simulink model "simulinkProject"  (R2023a)
settings: Solver=ode4  StartTime=0.0  StopTime=20  FixedStep=System.Ts  RelTol=1e-3
values from neighbouring files (symbols this model uses):
  b_end = 0.5*(K_end * (Lift.m + Tilt.m + Cylinder_3.m + Extension_2.m + Extension_1.m + Cylinder_4.m))^0.5    [project.m]
  b_end_1 = 0.5*(K_end_1 * (Lift.m + Pillar.m + Cylinder.m + Tilt.m + Cylinder_4.m + Cylinder_3.m + Extension_1.m + Extension_2.m))^0.5    [project.m]
  b_end_3 = 0.5*(K_end_3 * (Tilt.m + Extension_2.m + Extension_1.m + Cylinder_4.m))^0.5    [project.m]
  b_end_4 = 0.5*(K_end_4 * (Extension_2.m + Extension_1.m))^0.5    [project.m]
  K_end = p_max / delta_x    [project.m]
  K_end_1 = p_max_1 / delta_x_1    [project.m]
  K_end_3 = p_max_3 / delta_x_3    [project.m]
  K_end_4 = p_max_4 / delta_x_4    [project.m]
  Offset = 0.92    [project.m]
  Offset_1 = 0.72    [project.m]
  Offset_4 = 2.640    (= 2.64)    [project.m]
undefined symbols (not defined in the file or in its folder): Cylinder, Cylinder_1, Cylinder_3, Cylinder_4, Extension_1, fabs, Fourbar_1, Fourbar_2, Lift, Pillar, Pinion, Piston, Piston_3, Piston_4, sgn, System, System_1, System_3, System_4, Tilt, Valve, Valve_1, Valve_3, Valve_4, X, Y, Z
libraries: sm_lib x71, nesl_utility x27, TcTargetLib x1
(part 2 of 4)

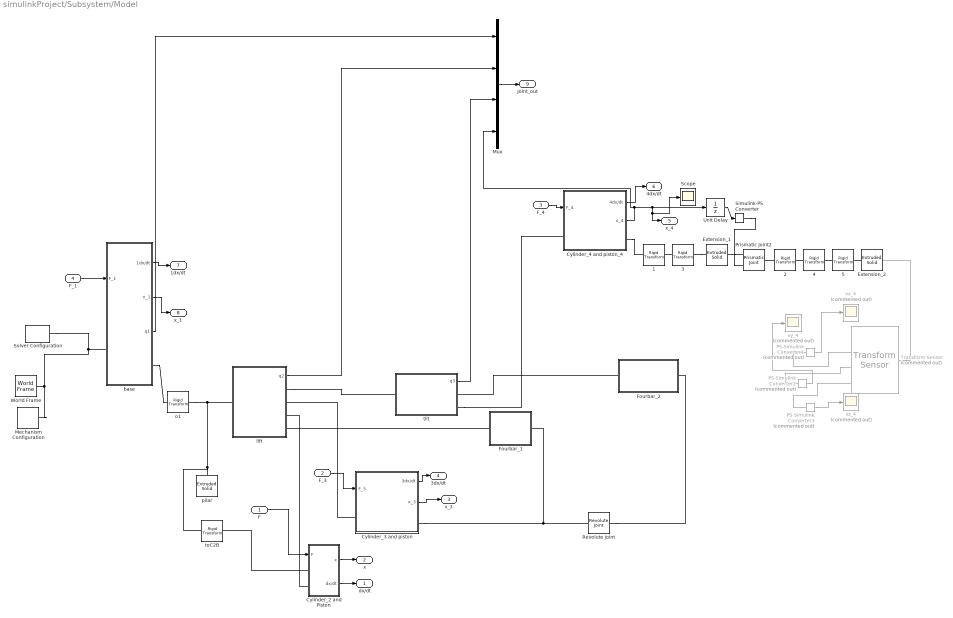
== system simulinkProject/Subsystem/Model ==
  F : Inport
  F_3 : Inport  Port=2
  F_4 : Inport  Port=3
  F_1 : Inport  Port=4
  1 : sm_lib/Frames and Transforms/Rigid Transform  TranslationMethod=None  TranslationStandardOffset=-0.2  TranslationStandardOffsetUnits=m  TranslationStandardAxis=+X  TranslationCartesianOffset=[0 0 -0.177]  TranslationCartesianOffsetUnits=m  TranslationROffset=0  TranslationROffsetUnits=m  TranslationZOffset=0  TranslationZOffsetUnits=m  TranslationThetaOffset=0  TranslationThetaOffsetUnits=deg  RotationMethod=StandardAxis  RotationAngleUnits=deg  RotationStandardAxis=-Y  RotationAngle=90.0  RotationArbitraryAxis=[0 0 1]  FollAlignAxisA=+X  BaseAlignAxisA=+Y  FollAlignAxisB=+Y  BaseAlignAxisB=+Z  RotationSequenceAxes=FollowerAxes  RotationSequence=XYX  RotationSequenceAngles=[0 0 0]  RotationSequenceAnglesUnits=deg  RotationMatrix=[1 0 0; 0 1 0; 0 0 1]  Quaternion=[1 0 0 0]
  2 : sm_lib/Frames and Transforms/Rigid Transform  TranslationMethod=None  TranslationStandardOffset=-0.5  TranslationStandardOffsetUnits=m  TranslationStandardAxis=-Z  TranslationCartesianOffset=[0 0 -0.177]  TranslationCartesianOffsetUnits=m  TranslationROffset=0  TranslationROffsetUnits=m  TranslationZOffset=0  TranslationZOffsetUnits=m  TranslationThetaOffset=0  TranslationThetaOffsetUnits=deg  RotationMethod=None  RotationAngleUnits=deg  RotationStandardAxis=+Y  RotationAngle=90.0  RotationArbitraryAxis=[0 0 1]  FollAlignAxisA=+X  BaseAlignAxisA=+Y  FollAlignAxisB=+Y  BaseAlignAxisB=+Z  RotationSequenceAxes=FollowerAxes  RotationSequence=XYX  RotationSequenceAngles=[0 0 0]  RotationSequenceAnglesUnits=deg  RotationMatrix=[1 0 0; 0 1 0; 0 0 1]  Quaternion=[1 0 0 0]
  3 : sm_lib/Frames and Transforms/Rigid Transform  TranslationMethod=None  TranslationStandardOffset=-0.2  TranslationStandardOffsetUnits=m  TranslationStandardAxis=+X  TranslationCartesianOffset=[0 0 -0.177]  TranslationCartesianOffsetUnits=m  TranslationROffset=0  TranslationROffsetUnits=m  TranslationZOffset=0  TranslationZOffsetUnits=m  TranslationThetaOffset=0  TranslationThetaOffsetUnits=deg  RotationMethod=StandardAxis  RotationAngleUnits=deg  RotationStandardAxis=-X  RotationAngle=90.0  RotationArbitraryAxis=[0 0 1]  FollAlignAxisA=+X  BaseAlignAxisA=+Y  FollAlignAxisB=+Y  BaseAlignAxisB=+Z  RotationSequenceAxes=FollowerAxes  RotationSequence=XYX  RotationSequenceAngles=[0 0 0]  RotationSequenceAnglesUnits=deg  RotationMatrix=[1 0 0; 0 1 0; 0 0 1]  Quaternion=[1 0 0 0]
  4 : sm_lib/Frames and Transforms/Rigid Transform  TranslationMethod=None  TranslationStandardOffset=-0.2  TranslationStandardOffsetUnits=m  TranslationStandardAxis=+X  TranslationCartesianOffset=[0 0 -0.177]  TranslationCartesianOffsetUnits=m  TranslationROffset=0  TranslationROffsetUnits=m  TranslationZOffset=0  TranslationZOffsetUnits=m  TranslationThetaOffset=0  TranslationThetaOffsetUnits=deg  RotationMethod=StandardAxis  RotationAngleUnits=deg  RotationStandardAxis=+X  RotationAngle=90.0  RotationArbitraryAxis=[0 0 1]  FollAlignAxisA=+X  BaseAlignAxisA=+Y  FollAlignAxisB=+Y  BaseAlignAxisB=+Z  RotationSequenceAxes=FollowerAxes  RotationSequence=XYX  RotationSequenceAngles=[0 0 0]  RotationSequenceAnglesUnits=deg  RotationMatrix=[1 0 0; 0 1 0; 0 0 1]  Quaternion=[1 0 0 0]
  5 : sm_lib/Frames and Transforms/Rigid Transform  TranslationMethod=None  TranslationStandardOffset=-0.2  TranslationStandardOffsetUnits=m  TranslationStandardAxis=+X  TranslationCartesianOffset=[0 0 -0.177]  TranslationCartesianOffsetUnits=m  TranslationROffset=0  TranslationROffsetUnits=m  TranslationZOffset=0  TranslationZOffsetUnits=m  TranslationThetaOffset=0  TranslationThetaOffsetUnits=deg  RotationMethod=StandardAxis  RotationAngleUnits=deg  RotationStandardAxis=-X  RotationAngle=90.0  RotationArbitraryAxis=[0 0 1]  FollAlignAxisA=+X  BaseAlignAxisA=+Y  FollAlignAxisB=+Y  BaseAlignAxisB=+Z  RotationSequenceAxes=FollowerAxes  RotationSequence=XYX  RotationSequenceAngles=[0 0 0]  RotationSequenceAnglesUnits=deg  RotationMatrix=[1 0 0; 0 1 0; 0 0 1]  Quaternion=[1 0 0 0]
  Cylinder_2 and Piston : Subsystem
  Cylinder_3 and piston : Subsystem
  Cylinder_4 and piston_4 : Subsystem
  Extension_1 : sm_lib/Body Elements/Extruded Solid  GraphicAmbientColor=[0.15 0.15 0.15 1.0]  BasedOnType=Mass  CenterOfMass=Extension_1.cm  CenterOfMassUnits=m  GraphicDiffuseColor=[0.0 0.6 0.6]  ExportConvexHullGeometry=off  ExtrusionCrossSection=Extension_1.cs  ExtrusionCrossSectionUnits=m  Density=1000  DensityUnits=kg/m^3  DoExposeReferenceFrame=off  GraphicEmissiveColor=[0.0 0.0 0.0 1.0]  ExportEntireGeometry=off  ExtrusionLength=0.2  ExtrusionLengthUnits=m  ExtrusionType=General  SerializedFrames=<Frames><Frame><Id>Frame1</Id><Value><Name>F1</Name><Origin><Source>GeometricFeature</Source><FeatureName>side surface 6</FeatureName></Origin><PrimaryAxis><DefinedDirection>+Z</DefinedDirection><Source>ReferenceFrame</Source><SourceDirection>+X</SourceDirection><FeatureName></FeatureName></PrimaryAxis><SecondaryAxis><DefinedDirection>+X</DefinedDirection><Source>ReferenceFrame</Source><SourceDirection>+Y</SourceDirection><FeatureName></FeatureName></SecondaryAxis></Value></Frame><Frame><Id>Frame2</Id><Value><Name>F2</Name><Origin><Source>GeometricFeature</Source><FeatureName>side curve 3</FeatureName></Origin><PrimaryAxis><DefinedDirection>+Z</DefinedDirection><Source>ReferenceFrame</Source><SourceDirection>+Z</SourceDirection><FeatureName></FeatureName></PrimaryAxis><SecondaryAxis><DefinedDirection>+X</DefinedDirection><Source>ReferenceFrame</Source><SourceDirection>+X</SourceDirection><FeatureName></FeatureName></SecondaryAxis></Value></Frame></Frames>  MarkerShape=Sphere  MarkerSize=10  GraphicType=FromGeometry  InertiaType=CalculateFromGeometry  Mass=Extension_1.m  MassUnits=kg  MomentsOfInertia=[1 1 1]  MomentsOfInertiaUnits=kg*m^2  PolygonNumSides=3  GraphicOpacity=1.0  PolygonOuterRadius=1  PolygonOuterRadiusUnits=m  ProductsOfInertia=[0 0 0]  ProductsOfInertiaUnits=kg*m^2  GraphicShininess=75  GraphicSpecularColor=[0.5 0.5 0.5 1.0]  GraphicVisPropType=SimpleVisualProperties
  Extension_2 : sm_lib/Body Elements/Extruded Solid  GraphicAmbientColor=[0.15 0.15 0.15 1.0]  BasedOnType=Mass  CenterOfMass=Extension_1.cm  CenterOfMassUnits=m  GraphicDiffuseColor=[0.2 0.0 0.4]  ExportConvexHullGeometry=off  ExtrusionCrossSection=Extension_1.cs  ExtrusionCrossSectionUnits=m  Density=1000  DensityUnits=kg/m^3  DoExposeReferenceFrame=off  GraphicEmissiveColor=[0.0 0.0 0.0 1.0]  ExportEntireGeometry=off  ExtrusionLength=0.2  ExtrusionLengthUnits=m  ExtrusionType=General  SerializedFrames=<Frames><Frame><Id>Frame1</Id><Value><Name>F1</Name><Origin><Source>GeometricFeature</Source><FeatureName>side surface 6</FeatureName></Origin><PrimaryAxis><DefinedDirection>+Z</DefinedDirection><Source>ReferenceFrame</Source><SourceDirection>+X</SourceDirection><FeatureName></FeatureName></PrimaryAxis><SecondaryAxis><DefinedDirection>+X</DefinedDirection><Source>ReferenceFrame</Source><SourceDirection>+Y</SourceDirection><FeatureName></FeatureName></SecondaryAxis></Value></Frame><Frame><Id>Frame2</Id><Value><Name>F2</Name><Origin><Source>GeometricFeature</Source><FeatureName>side curve 3</FeatureName></Origin><PrimaryAxis><DefinedDirection>+Z</DefinedDirection><Source>ReferenceFrame</Source><SourceDirection>+Z</SourceDirection><FeatureName></FeatureName></PrimaryAxis><SecondaryAxis><DefinedDirection>+X</DefinedDirection><Source>ReferenceFrame</Source><SourceDirection>+X</SourceDirection><FeatureName></FeatureName></SecondaryAxis></Value></Frame></Frames>  MarkerShape=Sphere  MarkerSize=10  GraphicType=FromGeometry  InertiaType=CalculateFromGeometry  Mass=Extension_1.m  MassUnits=kg  MomentsOfInertia=[1 1 1]  MomentsOfInertiaUnits=kg*m^2  PolygonNumSides=3  GraphicOpacity=1.0  PolygonOuterRadius=1  PolygonOuterRadiusUnits=m  ProductsOfInertia=[0 0 0]  ProductsOfInertiaUnits=kg*m^2  GraphicShininess=75  GraphicSpecularColor=[0.5 0.5 0.5 1.0]  GraphicVisPropType=SimpleVisualProperties
  Fourbar_1 : Subsystem
  Fourbar_2 : Subsystem
  Mechanism Configuration : sm_lib/Utilities/Mechanism Configuration  UniformGravity=Constant  GravityVector=[0 0 -9.80665]  GravityVectorUnits=m/s^2  LinearizationDelta=0.001  JointModeTransitionNonlinearIterations=2
  Mux : Mux
  PS-Simulink Converter1 : nesl_utility/PS-Simulink Converter  Commented=on  PhysicalDomain=network_engine_domain  SubClassName=ps_output  LeftPortType=input  RightPortType=output  PseudoPeriodic=off  Frequencies=[]  VectorFormat=inherit  Unit=inherit  AffineConversion=off
  PS-Simulink Converter2 : nesl_utility/PS-Simulink Converter  Commented=on  PhysicalDomain=network_engine_domain  SubClassName=ps_output  LeftPortType=input  RightPortType=output  PseudoPeriodic=off  Frequencies=[]  VectorFormat=inherit  Unit=inherit  AffineConversion=off
  PS-Simulink Converter3 : nesl_utility/PS-Simulink Converter  Commented=on  PhysicalDomain=network_engine_domain  SubClassName=ps_output  LeftPortType=input  RightPortType=output  PseudoPeriodic=off  Frequencies=[]  VectorFormat=inherit  Unit=inherit  AffineConversion=off
  Prismatic Joint2 : sm_lib/Joints/Prismatic Joint  JointMode=Normal  SenseConstraintForce=off  SenseConstraintForceX=off  SenseConstraintForceY=off  SenseConstraintForceZ=off  SenseConstraintTorque=off  SenseConstraintTorqueX=off  SenseConstraintTorqueY=off  SenseConstraintTorqueZ=off  SenseTotalForce=off  SenseTotalForceX=off  SenseTotalForceY=off  SenseTotalForceZ=off  SenseTotalTorque=off  SenseTotalTorqueX=off  SenseTotalTorqueY=off  SenseTotalTorqueZ=off  CompositeWrenchDir=FollowerOnBase  CompositeWrenchFrame=BaseFrame  EquilibriumPosition=0  EquilibriumPositionUnits=m  SpringStiffness=0  SpringStiffnessUnits=N/m  DampingCoefficient=0  DampingCoefficientUnits=N/(m/s)  TorqueActuationMode=ComputedTorque  MotionActuationMode=InputMotion  SensePosition=off  SenseVelocity=off  SenseAcceleration=off  SenseTorqueForce=off  SenseLowerLimitTorqueForce=off  SenseUpperLimitTorqueForce=off  LowerLimitSpecify=off  LowerLimitBound=-1  LowerLimitBoundUnits=m  LowerLimitStiffness=1e6  LowerLimitStiffnessUnits=N/m  LowerLimitDamping=1e3  LowerLimitDampingUnits=N/(m/s)  LowerLimitTransitionRegionWidth=1e-4  LowerLimitTransitionRegionWidthUnits=m  UpperLimitSpecify=off  UpperLimitBound=1  UpperLimitBoundUnits=m  UpperLimitStiffness=1e6  UpperLimitStiffnessUnits=N/m  UpperLimitDamping=1e3  UpperLimitDampingUnits=N/(m/s)  UpperLimitTransitionRegionWidth=1e-4  UpperLimitTransitionRegionWidthUnits=m  PositionTargetSpecify=on  PositionTargetPriority=High  PositionTargetValue=0.2  PositionTargetValueUnits=m  VelocityTargetSpecify=off  VelocityTargetPriority=High  VelocityTargetValue=0  VelocityTargetValueUnits=m/s
  Revolute Joint : sm_lib/Joints/Revolute Joint  JointMode=Normal  SenseConstraintForce=off  SenseConstraintForceX=off  SenseConstraintForceY=off  SenseConstraintForceZ=off  SenseConstraintTorque=off  SenseConstraintTorqueX=off  SenseConstraintTorqueY=off  SenseConstraintTorqueZ=off  SenseTotalForce=off  SenseTotalForceX=off  SenseTotalForceY=off  SenseTotalForceZ=off  SenseTotalTorque=off  SenseTotalTorqueX=off  SenseTotalTorqueY=off  SenseTotalTorqueZ=off  CompositeWrenchDir=FollowerOnBase  CompositeWrenchFrame=BaseFrame  EquilibriumPosition=0  EquilibriumPositionUnits=deg  SpringStiffness=0  SpringStiffnessUnits=N*m/deg  DampingCoefficient=0  DampingCoefficientUnits=N*m/(deg/s)  TorqueActuationMode=NoTorque  MotionActuationMode=ComputedMotion  SensePosition=off  SenseVelocity=off  SenseAcceleration=off  SenseTorqueForce=off  SenseLowerLimitTorqueForce=off  SenseUpperLimitTorqueForce=off  LowerLimitSpecify=off  LowerLimitBound=-90  LowerLimitBoundUnits=deg  LowerLimitStiffness=1e4  LowerLimitStiffnessUnits=N*m/deg  LowerLimitDamping=10  LowerLimitDampingUnits=N*m/(deg/s)  LowerLimitTransitionRegionWidth=0.1  LowerLimitTransitionRegionWidthUnits=deg  UpperLimitSpecify=off  UpperLimitBound=90  UpperLimitBoundUnits=deg  UpperLimitStiffness=1e4  UpperLimitStiffnessUnits=N*m/deg  UpperLimitDamping=10  UpperLimitDampingUnits=N*m/(deg/s)  UpperLimitTransitionRegionWidth=0.1  UpperLimitTransitionRegionWidthUnits=deg  PositionTargetSpecify=off  PositionTargetPriority=Low  PositionTargetValue=-80  PositionTargetValueUnits=deg  VelocityTargetSpecify=off  VelocityTargetPriority=High  VelocityTargetValue=0  VelocityTargetValueUnits=deg/s
  Scope : Scope
  Simulink-PS Converter : nesl_utility/Simulink-PS Converter  PhysicalDomain=network_engine_domain  SubClassName=ps_input  LeftPortType=input  RightPortType=output  PseudoPeriodic=off  Frequencies=[]  NoiseDistribution=none  NoiseParameters=[]  Unit=1  AffineConversion=off  FilteringAndDerivatives=filter  SimscapeFilterOrder=2  InputFilterTimeConstant=0.005  UdotUserProvided=0
  Solver Configuration : nesl_utility/Solver Configuration  PhysicalDomain=network_engine_domain  SubClassName=solver  LeftPortType=input  RightPortType=generic  Tones=[]  Harmonics=[]  SimulateNoise=off  Profile=off  UseLocalSampling=off  EnableSwitchedLinearOptims=on  FrequencyDomain=off  UseCCode=off  RelTol=0.001  AbsTol=0.001  MinStep=1e-09  ToWorkspace=off  RevertToSquareIcSolve=off  NumHomotopyIterations=100  PhasorMode=off  PhasorModeNumHarmonics=1  ConsistencySolver=NEWTON_XTOL_AFTER_FTOL  IndexReductionMethod=DerivativeReplacement  DoDC=off  ResidualTolerance=1e-09  ConsistencyTolSource=GLOBAL  ConsistencyAbsTol=0.001  ConsistencyRelTol=0.001  ConsistencyTolFactor=0.001  UseLocalSolver=off  LocalSolverChoice=NE_BACKWARD_EULER_ADVANCER  ResolveIndetEquations=on  FunctionEvalNumThread=1  LocalSolverSampleTime=0.001  DoFixedCost=off  MaxNonlinIter=3  MaxModeIter=2  ComputeImpulses=off  ImpulseIterations=2  LinearAlgebra=auto  LinearAlgebraNumThread=0  EquationFormulation=NE_TIME_EF  DelaysMemoryBudget=1024  AutomaticFiltering=on  FilteringTimeConstant=0.001  PartitionStorageMethod=AS_NEEDED  PartitionMemoryBudget=1024  PartitionMethod=ROBUST
  Transform Sensor : sm_lib/Frames and Transforms/Transform Sensor  Commented=on  MeasurementFrame=World  RotationSequence=XYX  SenseAngle=off  SenseAxis=off  SenseQ=off  SenseR=off  SenseRotationSequence=off  SenseOmegaX=off  SenseOmegaY=off  SenseOmegaZ=off  SenseQDot=off  SenseRDot=off  SenseRotationSequenceDot=off  SenseAlphaX=off  SenseAlphaY=off  SenseAlphaZ=off  SenseQDDot=off  SenseRDDot=off  SenseX=off  SenseY=off  SenseZ=off  SenseRad=off  SenseAzim=off  SenseDist=off  SenseInc=off  SenseXDot=on  SenseYDot=on  SenseZDot=on  SenseRadDot=off  SenseAzimDot=off  SenseDistDot=off  SenseIncDot=off  SenseXDDot=off  SenseYDDot=off  SenseZDDot=off  SenseRadDDot=off  SenseAzimDDot=off  SenseDistDDot=off  SenseIncDDot=off
  Unit Delay : UnitDelay  InitialCondition=0.2  SampleTime=-1  HasFrameUpgradeWarning=on
  World Frame : sm_lib/Frames and Transforms/World Frame
  base : Subsystem
  lift : Subsystem
  o1 : sm_lib/Frames and Transforms/Rigid Transform  TranslationMethod=None  TranslationStandardOffset=0  TranslationStandardOffsetUnits=m  TranslationStandardAxis=+Z  TranslationCartesianOffset=[0 0 0]  TranslationCartesianOffsetUnits=m  TranslationROffset=0  TranslationROffsetUnits=m  TranslationZOffset=0  TranslationZOffsetUnits=m  TranslationThetaOffset=0  TranslationThetaOffsetUnits=deg  RotationMethod=StandardAxis  RotationAngleUnits=deg  RotationStandardAxis=+X  RotationAngle=90.0  RotationArbitraryAxis=[0 0 1]  FollAlignAxisA=+X  BaseAlignAxisA=+Y  FollAlignAxisB=+Y  BaseAlignAxisB=+Z  RotationSequenceAxes=FollowerAxes  RotationSequence=XYX  RotationSequenceAngles=[0 0 0]  RotationSequenceAnglesUnits=deg  RotationMatrix=[1 0 0; 0 1 0; 0 0 1]  Quaternion=[1 0 0 0]
  pilar : sm_lib/Body Elements/Extruded Solid  GraphicAmbientColor=[0.15 0.15 0.15 1.0]  BasedOnType=Density  CenterOfMass=Pillar.cm  CenterOfMassUnits=m  GraphicDiffuseColor=Pillar.rgb  ExportConvexHullGeometry=off  ExtrusionCrossSection=Pillar.cs  ExtrusionCrossSectionUnits=m  Density=1000  DensityUnits=kg/m^3  DoExposeReferenceFrame=on  GraphicEmissiveColor=[0.0 0.0 0.0 1.0]  ExportEntireGeometry=off  ExtrusionLength=Pillar.l  ExtrusionLengthUnits=m  ExtrusionType=General  SerializedFrames=<Frames/>  MarkerShape=Sphere  MarkerSize=10  GraphicType=FromGeometry  InertiaType=Custom  Mass=Pillar.m  MassUnits=kg  MomentsOfInertia=[1 1 1]  MomentsOfInertiaUnits=kg*m^2  PolygonNumSides=3  GraphicOpacity=1.0  PolygonOuterRadius=1  PolygonOuterRadiusUnits=m  ProductsOfInertia=[0 0 0]  ProductsOfInertiaUnits=kg*m^2  GraphicShininess=75  GraphicSpecularColor=[0.5 0.5 0.5 1.0]  GraphicVisPropType=SimpleVisualProperties
  tilt : Subsystem
  toC2B : sm_lib/Frames and Transforms/Rigid Transform  TranslationMethod=Cartesian  TranslationStandardOffset=0  TranslationStandardOffsetUnits=m  TranslationStandardAxis=+Z  TranslationCartesianOffset=Piston.pos  TranslationCartesianOffsetUnits=m  TranslationROffset=0  TranslationROffsetUnits=m  TranslationZOffset=0  TranslationZOffsetUnits=m  TranslationThetaOffset=0  TranslationThetaOffsetUnits=deg  RotationMethod=None  RotationAngleUnits=deg  RotationStandardAxis=+Z  RotationAngle=90.0  RotationArbitraryAxis=[0 0 1]  FollAlignAxisA=+X  BaseAlignAxisA=+Y  FollAlignAxisB=+Y  BaseAlignAxisB=+Z  RotationSequenceAxes=FollowerAxes  RotationSequence=XYX  RotationSequenceAngles=[0 0 0]  RotationSequenceAnglesUnits=deg  RotationMatrix=[1 0 0; 0 1 0; 0 0 1]  Quaternion=[1 0 0 0]
  vx_4 : Scope  Commented=on
  vy_4 : Scope  Commented=on
  vz_4 : Scope  Commented=on
  dx/dt : Outport
  x : Outport  Port=2
  x_3 : Outport  Port=3
  3dx/dt : Outport  Port=4
  x_4 : Outport  Port=5
  4dx/dt : Outport  Port=6
  1dx/dt : Outport  Port=7
  x_1 : Outport  Port=8
  Joint_out : Outport  Port=9
  wires:
  F/1 -> Cylinder_2 and Piston/1(F)
  Cylinder_2 and Piston/1(x) -> x/1
  Cylinder_2 and Piston/2(dx/dt) -> dx/dt/1
  F_3/1 -> Cylinder_3 and piston/1(F_3)
  Cylinder_3 and piston/1(3dx/dt) -> 3dx/dt/1
  F_4/1 -> Cylinder_4 and piston_4/1(F_4)
  Unit Delay/1 -> Simulink-PS Converter/1
  Cylinder_4 and piston_4/1(4dx/dt) -> 4dx/dt/1
  Cylinder_4 and piston_4/2(x_4) -> Mux/4, Unit Delay/1, Scope/1, x_4/1
  Cylinder_3 and piston/2(x_3) -> x_3/1
  F_1/1 -> base/1(F_1)
  base/2(x_1) -> x_1/1
  base/1(1dx/dt) -> 1dx/dt/1
  PS-Simulink Converter1/1 -> vx_4/1
  PS-Simulink Converter3/1 -> vz_4/1
  PS-Simulink Converter2/1 -> vy_4/1
  Mux/1 -> Joint_out/1
  tilt/1(q3) -> Mux/3
  lift/1(q2) -> Mux/2
  base/3(q1) -> Mux/1
  connections:
  World Frame/RConn1 -- Mechanism Configuration/RConn1 -- Solver Configuration/RConn1 -- base/LConn1
  pilar/RConn1 -- o1/RConn1 -- lift/LConn1 -- toC2B/LConn1
  Cylinder_2 and Piston/LConn1 -- toC2B/RConn1
  base/RConn1 -- o1/LConn1
  Cylinder_2 and Piston/LConn2 -- lift/RConn3
  lift/RConn1 -- tilt/LConn1
  Cylinder_3 and piston/LConn1 -- lift/RConn2
  tilt/RConn2 -- Cylinder_4 and piston_4/LConn1
  Fourbar_2/LConn1 -- tilt/RConn1
  Fourbar_1/LConn1 -- lift/RConn4
  Cylinder_3 and piston/RConn1 -- Fourbar_1/RConn1 -- Revolute Joint/LConn1
  Revolute Joint/RConn1 -- Fourbar_2/RConn1
  Simulink-PS Converter/RConn1 -- Prismatic Joint2/LConn2
  Extension_1/LConn1 -- Prismatic Joint2/LConn1
  Cylinder_4 and piston_4/RConn1 -- 1/LConn1
  3/LConn1 -- 1/RConn1
  3/RConn1 -- Extension_1/RConn1
  5/LConn1 -- 4/RConn1
  5/RConn1 -- Extension_2/LConn1
  2/RConn1 -- 4/LConn1
  2/LConn1 -- Prismatic Joint2/RConn1
  Transform Sensor/LConn1 -- Extension_2/RConn1
  PS-Simulink Converter1/LConn1 -- Transform Sensor/RConn2
  PS-Simulink Converter2/LConn1 -- Transform Sensor/RConn3
  PS-Simulink Converter3/LConn1 -- Transform Sensor/RConn4

== system simulinkProject/Subsystem/4//3 Servovalve_1/Orifice P->A ==
  dp : Inport
  u : Inport  Port=2
  Fcn : Fcn  Expr=u[2]*u[1]/2.0/sqrt(ptr)*(3-u[1]/ptr)
  Fcn1 : Fcn  Expr=(u(2)>=ptr)*u(1)+(u(2)<ptr)*u(3)
  Fcn2 : Fcn  Expr=sgn(u(1))
  Fcn3 : Fcn  Expr=fabs(u(1))
  Gain : Gain  Gain=K  SaturateOnIntegerOverflow=on  OutDataTypeStr=Inherit: Same as input  ParamDataTypeStr=Inherit: Same as input
  Math Function1 : Math  Operator=sqrt  SignedPower=on
  Mux : Mux  Inputs=2
  Mux1 : Mux  Inputs=3
  Product : Product  InputSameDT=on  SaturateOnIntegerOverflow=on  OutDataTypeStr=Inherit: Same as first input
  Product1 : Product  InputSameDT=on  SaturateOnIntegerOverflow=on  OutDataTypeStr=Inherit: Same as first input
  Saturation : Saturate  UpperLimit=inf  LowerLimit=0
  Q : Outport  InitialOutput=0  VectorParamsAs1DForOutWhenUnconnected=off
  wires:
  u/1 -> Saturation/1
  dp/1 -> Fcn3/1, Fcn2/1
  Fcn/1 -> Mux1/3
  Mux/1 -> Fcn/1
  Product/1 -> Mux1/1
  Math Function1/1 -> Product/1
  Fcn3/1 -> Mux/1, Mux1/2, Math Function1/1
  Saturation/1 -> Gain/1
  Gain/1 -> Product/2, Mux/2
  Mux1/1 -> Fcn1/1
  Fcn1/1 -> Product1/2
  Fcn2/1 -> Product1/1
  Product1/1 -> Q/1

== system simulinkProject/Subsystem/4//3 Servovalve_1/Orifice P->B ==
  dp : Inport
  u : Inport  Port=2
  Fcn : Fcn  Expr=u[2]*u[1]/2.0/sqrt(ptr)*(3-u[1]/ptr)
  Fcn1 : Fcn  Expr=(u(2)>=ptr)*u(1)+(u(2)<ptr)*u(3)
  Fcn2 : Fcn  Expr=sgn(u(1))
  Fcn3 : Fcn  Expr=fabs(u(1))
  Gain : Gain  Gain=K  SaturateOnIntegerOverflow=on  OutDataTypeStr=Inherit: Same as input  ParamDataTypeStr=Inherit: Same as input
  Math Function1 : Math  Operator=sqrt  SignedPower=on
  Mux : Mux  Inputs=2
  Mux1 : Mux  Inputs=3
  Product : Product  InputSameDT=on  SaturateOnIntegerOverflow=on  OutDataTypeStr=Inherit: Same as first input
  Product1 : Product  InputSameDT=on  SaturateOnIntegerOverflow=on  OutDataTypeStr=Inherit: Same as first input
  Saturation : Saturate  UpperLimit=inf  LowerLimit=0
  Q : Outport  InitialOutput=0  VectorParamsAs1DForOutWhenUnconnected=off
  wires:
  u/1 -> Saturation/1
  dp/1 -> Fcn3/1, Fcn2/1
  Fcn/1 -> Mux1/3
  Mux/1 -> Fcn/1
  Product/1 -> Mux1/1
  Math Function1/1 -> Product/1
  Fcn3/1 -> Mux/1, Mux1/2, Math Function1/1
  Saturation/1 -> Gain/1
  Gain/1 -> Product/2, Mux/2
  Mux1/1 -> Fcn1/1
  Fcn1/1 -> Product1/2
  Fcn2/1 -> Product1/1
  Product1/1 -> Q/1

== system simulinkProject/Subsystem/4//3 Servovalve_1/Orifice T->A ==
  dp : Inport
  u : Inport  Port=2
  Fcn : Fcn  Expr=u[2]*u[1]/2.0/sqrt(ptr)*(3-u[1]/ptr)
  Fcn1 : Fcn  Expr=(u(2)>=ptr)*u(1)+(u(2)<ptr)*u(3)
  Fcn2 : Fcn  Expr=sgn(u(1))
  Fcn3 : Fcn  Expr=fabs(u(1))
  Gain : Gain  Gain=K  SaturateOnIntegerOverflow=on  OutDataTypeStr=Inherit: Same as input  ParamDataTypeStr=Inherit: Same as input
  Math Function1 : Math  Operator=sqrt  SignedPower=on
  Mux : Mux  Inputs=2
  Mux1 : Mux  Inputs=3
  Product : Product  InputSameDT=on  SaturateOnIntegerOverflow=on  OutDataTypeStr=Inherit: Same as first input
  Product1 : Product  InputSameDT=on  SaturateOnIntegerOverflow=on  OutDataTypeStr=Inherit: Same as first input
  Saturation : Saturate  UpperLimit=inf  LowerLimit=0
  Q : Outport  InitialOutput=0  VectorParamsAs1DForOutWhenUnconnected=off
  wires:
  u/1 -> Saturation/1
  dp/1 -> Fcn3/1, Fcn2/1
  Fcn/1 -> Mux1/3
  Mux/1 -> Fcn/1
  Product/1 -> Mux1/1
  Math Function1/1 -> Product/1
  Fcn3/1 -> Mux/1, Mux1/2, Math Function1/1
  Saturation/1 -> Gain/1
  Gain/1 -> Product/2, Mux/2
  Mux1/1 -> Fcn1/1
  Fcn1/1 -> Product1/2
  Fcn2/1 -> Product1/1
  Product1/1 -> Q/1

== system simulinkProject/Subsystem/4//3 Servovalve_1/Orifice T->B ==
  dp : Inport
  u : Inport  Port=2
  Fcn : Fcn  Expr=u[2]*u[1]/2.0/sqrt(ptr)*(3-u[1]/ptr)
  Fcn1 : Fcn  Expr=(u(2)>=ptr)*u(1)+(u(2)<ptr)*u(3)
  Fcn2 : Fcn  Expr=sgn(u(1))
  Fcn3 : Fcn  Expr=fabs(u(1))
  Gain : Gain  Gain=K  SaturateOnIntegerOverflow=on  OutDataTypeStr=Inherit: Same as input  ParamDataTypeStr=Inherit: Same as input
  Math Function1 : Math  Operator=sqrt  SignedPower=on
  Mux : Mux  Inputs=2
  Mux1 : Mux  Inputs=3
  Product : Product  InputSameDT=on  SaturateOnIntegerOverflow=on  OutDataTypeStr=Inherit: Same as first input
  Product1 : Product  InputSameDT=on  SaturateOnIntegerOverflow=on  OutDataTypeStr=Inherit: Same as first input
  Saturation : Saturate  UpperLimit=inf  LowerLimit=0
  Q : Outport  InitialOutput=0  VectorParamsAs1DForOutWhenUnconnected=off
  wires:
  u/1 -> Saturation/1
  dp/1 -> Fcn3/1, Fcn2/1
  Fcn/1 -> Mux1/3
  Mux/1 -> Fcn/1
  Product/1 -> Mux1/1
  Math Function1/1 -> Product/1
  Fcn3/1 -> Mux/1, Mux1/2, Math Function1/1
  Saturation/1 -> Gain/1
  Gain/1 -> Product/2, Mux/2
  Mux1/1 -> Fcn1/1
  Fcn1/1 -> Product1/2
  Fcn2/1 -> Product1/1
  Product1/1 -> Q/1

== system simulinkProject/Subsystem/4//3 Servovalve_2/Orifice P->A ==
  dp : Inport
  u : Inport  Port=2
  Fcn : Fcn  Expr=u[2]*u[1]/2.0/sqrt(ptr)*(3-u[1]/ptr)
  Fcn1 : Fcn  Expr=(u(2)>=ptr)*u(1)+(u(2)<ptr)*u(3)
  Fcn2 : Fcn  Expr=sgn(u(1))
  Fcn3 : Fcn  Expr=fabs(u(1))
  Gain : Gain  Gain=K  SaturateOnIntegerOverflow=on  OutDataTypeStr=Inherit: Same as input  ParamDataTypeStr=Inherit: Same as input
  Math Function1 : Math  Operator=sqrt  SignedPower=on
  Mux : Mux  Inputs=2
  Mux1 : Mux  Inputs=3
  Product : Product  InputSameDT=on  SaturateOnIntegerOverflow=on  OutDataTypeStr=Inherit: Same as first input
  Product1 : Product  InputSameDT=on  SaturateOnIntegerOverflow=on  OutDataTypeStr=Inherit: Same as first input
  Saturation : Saturate  UpperLimit=inf  LowerLimit=0
  Q : Outport  InitialOutput=0  VectorParamsAs1DForOutWhenUnconnected=off
  wires:
  u/1 -> Saturation/1
  dp/1 -> Fcn3/1, Fcn2/1
  Fcn/1 -> Mux1/3
  Mux/1 -> Fcn/1
  Product/1 -> Mux1/1
  Math Function1/1 -> Product/1
  Fcn3/1 -> Mux/1, Mux1/2, Math Function1/1
  Saturation/1 -> Gain/1
  Gain/1 -> Product/2, Mux/2
  Mux1/1 -> Fcn1/1
  Fcn1/1 -> Product1/2
  Fcn2/1 -> Product1/1
  Product1/1 -> Q/1

== system simulinkProject/Subsystem/4//3 Servovalve_2/Orifice P->B ==
  dp : Inport
  u : Inport  Port=2
  Fcn : Fcn  Expr=u[2]*u[1]/2.0/sqrt(ptr)*(3-u[1]/ptr)
  Fcn1 : Fcn  Expr=(u(2)>=ptr)*u(1)+(u(2)<ptr)*u(3)
  Fcn2 : Fcn  Expr=sgn(u(1))
  Fcn3 : Fcn  Expr=fabs(u(1))
  Gain : Gain  Gain=K  SaturateOnIntegerOverflow=on  OutDataTypeStr=Inherit: Same as input  ParamDataTypeStr=Inherit: Same as input
  Math Function1 : Math  Operator=sqrt  SignedPower=on
  Mux : Mux  Inputs=2
  Mux1 : Mux  Inputs=3
  Product : Product  InputSameDT=on  SaturateOnIntegerOverflow=on  OutDataTypeStr=Inherit: Same as first input
  Product1 : Product  InputSameDT=on  SaturateOnIntegerOverflow=on  OutDataTypeStr=Inherit: Same as first input
  Saturation : Saturate  UpperLimit=inf  LowerLimit=0
  Q : Outport  InitialOutput=0  VectorParamsAs1DForOutWhenUnconnected=off
  wires:
  u/1 -> Saturation/1
  dp/1 -> Fcn3/1, Fcn2/1
  Fcn/1 -> Mux1/3
  Mux/1 -> Fcn/1
  Product/1 -> Mux1/1
  Math Function1/1 -> Product/1
  Fcn3/1 -> Mux/1, Mux1/2, Math Function1/1
  Saturation/1 -> Gain/1
  Gain/1 -> Product/2, Mux/2
  Mux1/1 -> Fcn1/1
  Fcn1/1 -> Product1/2
  Fcn2/1 -> Product1/1
  Product1/1 -> Q/1

== system simulinkProject/Subsystem/4//3 Servovalve_2/Orifice T->A ==
  dp : Inport
  u : Inport  Port=2
  Fcn : Fcn  Expr=u[2]*u[1]/2.0/sqrt(ptr)*(3-u[1]/ptr)
  Fcn1 : Fcn  Expr=(u(2)>=ptr)*u(1)+(u(2)<ptr)*u(3)
  Fcn2 : Fcn  Expr=sgn(u(1))
  Fcn3 : Fcn  Expr=fabs(u(1))
  Gain : Gain  Gain=K  SaturateOnIntegerOverflow=on  OutDataTypeStr=Inherit: Same as input  ParamDataTypeStr=Inherit: Same as input
  Math Function1 : Math  Operator=sqrt  SignedPower=on
  Mux : Mux  Inputs=2
  Mux1 : Mux  Inputs=3
  Product : Product  InputSameDT=on  SaturateOnIntegerOverflow=on  OutDataTypeStr=Inherit: Same as first input
  Product1 : Product  InputSameDT=on  SaturateOnIntegerOverflow=on  OutDataTypeStr=Inherit: Same as first input
  Saturation : Saturate  UpperLimit=inf  LowerLimit=0
  Q : Outport  InitialOutput=0  VectorParamsAs1DForOutWhenUnconnected=off
  wires:
  u/1 -> Saturation/1
  dp/1 -> Fcn3/1, Fcn2/1
  Fcn/1 -> Mux1/3
  Mux/1 -> Fcn/1
  Product/1 -> Mux1/1
  Math Function1/1 -> Product/1
  Fcn3/1 -> Mux/1, Mux1/2, Math Function1/1
  Saturation/1 -> Gain/1
  Gain/1 -> Product/2, Mux/2
  Mux1/1 -> Fcn1/1
  Fcn1/1 -> Product1/2
  Fcn2/1 -> Product1/1
  Product1/1 -> Q/1

== system simulinkProject/Subsystem/4//3 Servovalve_2/Orifice T->B ==
  dp : Inport
  u : Inport  Port=2
  Fcn : Fcn  Expr=u[2]*u[1]/2.0/sqrt(ptr)*(3-u[1]/ptr)
  Fcn1 : Fcn  Expr=(u(2)>=ptr)*u(1)+(u(2)<ptr)*u(3)
  Fcn2 : Fcn  Expr=sgn(u(1))
  Fcn3 : Fcn  Expr=fabs(u(1))
  Gain : Gain  Gain=K  SaturateOnIntegerOverflow=on  OutDataTypeStr=Inherit: Same as input  ParamDataTypeStr=Inherit: Same as input
  Math Function1 : Math  Operator=sqrt  SignedPower=on
  Mux : Mux  Inputs=2
  Mux1 : Mux  Inputs=3
  Product : Product  InputSameDT=on  SaturateOnIntegerOverflow=on  OutDataTypeStr=Inherit: Same as first input
  Product1 : Product  InputSameDT=on  SaturateOnIntegerOverflow=on  OutDataTypeStr=Inherit: Same as first input
  Saturation : Saturate  UpperLimit=inf  LowerLimit=0
  Q : Outport  InitialOutput=0  VectorParamsAs1DForOutWhenUnconnected=off
  wires:
  u/1 -> Saturation/1
  dp/1 -> Fcn3/1, Fcn2/1
  Fcn/1 -> Mux1/3
  Mux/1 -> Fcn/1
  Product/1 -> Mux1/1
  Math Function1/1 -> Product/1
  Fcn3/1 -> Mux/1, Mux1/2, Math Function1/1
  Saturation/1 -> Gain/1
  Gain/1 -> Product/2, Mux/2
  Mux1/1 -> Fcn1/1
  Fcn1/1 -> Product1/2
  Fcn2/1 -> Product1/1
  Product1/1 -> Q/1

== system simulinkProject/Subsystem/4//3 Servovalve_3/Orifice P->A ==
  dp : Inport
  u : Inport  Port=2
  Fcn : Fcn  Expr=u[2]*u[1]/2.0/sqrt(ptr)*(3-u[1]/ptr)
  Fcn1 : Fcn  Expr=(u(2)>=ptr)*u(1)+(u(2)<ptr)*u(3)
  Fcn2 : Fcn  Expr=sgn(u(1))
  Fcn3 : Fcn  Expr=fabs(u(1))
  Gain : Gain  Gain=K  SaturateOnIntegerOverflow=on  OutDataTypeStr=Inherit: Same as input  ParamDataTypeStr=Inherit: Same as input
  Math Function1 : Math  Operator=sqrt  SignedPower=on
  Mux : Mux  Inputs=2
  Mux1 : Mux  Inputs=3
  Product : Product  InputSameDT=on  SaturateOnIntegerOverflow=on  OutDataTypeStr=Inherit: Same as first input
  Product1 : Product  InputSameDT=on  SaturateOnIntegerOverflow=on  OutDataTypeStr=Inherit: Same as first input
  Saturation : Saturate  UpperLimit=inf  LowerLimit=0
  Q : Outport  InitialOutput=0  VectorParamsAs1DForOutWhenUnconnected=off
  wires:
  u/1 -> Saturation/1
  dp/1 -> Fcn3/1, Fcn2/1
  Fcn/1 -> Mux1/3
  Mux/1 -> Fcn/1
  Product/1 -> Mux1/1
  Math Function1/1 -> Product/1
  Fcn3/1 -> Mux/1, Mux1/2, Math Function1/1
  Saturation/1 -> Gain/1
  Gain/1 -> Product/2, Mux/2
  Mux1/1 -> Fcn1/1
  Fcn1/1 -> Product1/2
  Fcn2/1 -> Product1/1
  Product1/1 -> Q/1

== system simulinkProject/Subsystem/4//3 Servovalve_3/Orifice P->B ==
  dp : Inport
  u : Inport  Port=2
  Fcn : Fcn  Expr=u[2]*u[1]/2.0/sqrt(ptr)*(3-u[1]/ptr)
  Fcn1 : Fcn  Expr=(u(2)>=ptr)*u(1)+(u(2)<ptr)*u(3)
  Fcn2 : Fcn  Expr=sgn(u(1))
  Fcn3 : Fcn  Expr=fabs(u(1))
  Gain : Gain  Gain=K  SaturateOnIntegerOverflow=on  OutDataTypeStr=Inherit: Same as input  ParamDataTypeStr=Inherit: Same as input
  Math Function1 : Math  Operator=sqrt  SignedPower=on
  Mux : Mux  Inputs=2
  Mux1 : Mux  Inputs=3
  Product : Product  InputSameDT=on  SaturateOnIntegerOverflow=on  OutDataTypeStr=Inherit: Same as first input
  Product1 : Product  InputSameDT=on  SaturateOnIntegerOverflow=on  OutDataTypeStr=Inherit: Same as first input
  Saturation : Saturate  UpperLimit=inf  LowerLimit=0
  Q : Outport  InitialOutput=0  VectorParamsAs1DForOutWhenUnconnected=off
  wires:
  u/1 -> Saturation/1
  dp/1 -> Fcn3/1, Fcn2/1
  Fcn/1 -> Mux1/3
  Mux/1 -> Fcn/1
  Product/1 -> Mux1/1
  Math Function1/1 -> Product/1
  Fcn3/1 -> Mux/1, Mux1/2, Math Function1/1
  Saturation/1 -> Gain/1
  Gain/1 -> Product/2, Mux/2
  Mux1/1 -> Fcn1/1
  Fcn1/1 -> Product1/2
  Fcn2/1 -> Product1/1
  Product1/1 -> Q/1

== system simulinkProject/Subsystem/4//3 Servovalve_3/Orifice T->A ==
  dp : Inport
  u : Inport  Port=2
  Fcn : Fcn  Expr=u[2]*u[1]/2.0/sqrt(ptr)*(3-u[1]/ptr)
  Fcn1 : Fcn  Expr=(u(2)>=ptr)*u(1)+(u(2)<ptr)*u(3)
  Fcn2 : Fcn  Expr=sgn(u(1))
  Fcn3 : Fcn  Expr=fabs(u(1))
  Gain : Gain  Gain=K  SaturateOnIntegerOverflow=on  OutDataTypeStr=Inherit: Same as input  ParamDataTypeStr=Inherit: Same as input
  Math Function1 : Math  Operator=sqrt  SignedPower=on
  Mux : Mux  Inputs=2
  Mux1 : Mux  Inputs=3
  Product : Product  InputSameDT=on  SaturateOnIntegerOverflow=on  OutDataTypeStr=Inherit: Same as first input
  Product1 : Product  InputSameDT=on  SaturateOnIntegerOverflow=on  OutDataTypeStr=Inherit: Same as first input
  Saturation : Saturate  UpperLimit=inf  LowerLimit=0
  Q : Outport  InitialOutput=0  VectorParamsAs1DForOutWhenUnconnected=off
  wires:
  u/1 -> Saturation/1
  dp/1 -> Fcn3/1, Fcn2/1
  Fcn/1 -> Mux1/3
  Mux/1 -> Fcn/1
  Product/1 -> Mux1/1
  Math Function1/1 -> Product/1
  Fcn3/1 -> Mux/1, Mux1/2, Math Function1/1
  Saturation/1 -> Gain/1
  Gain/1 -> Product/2, Mux/2
  Mux1/1 -> Fcn1/1
  Fcn1/1 -> Product1/2
  Fcn2/1 -> Product1/1
  Product1/1 -> Q/1

== system simulinkProject/Subsystem/4//3 Servovalve_3/Orifice T->B ==
  dp : Inport
  u : Inport  Port=2
  Fcn : Fcn  Expr=u[2]*u[1]/2.0/sqrt(ptr)*(3-u[1]/ptr)
  Fcn1 : Fcn  Expr=(u(2)>=ptr)*u(1)+(u(2)<ptr)*u(3)
  Fcn2 : Fcn  Expr=sgn(u(1))
  Fcn3 : Fcn  Expr=fabs(u(1))
  Gain : Gain  Gain=K  SaturateOnIntegerOverflow=on  OutDataTypeStr=Inherit: Same as input  ParamDataTypeStr=Inherit: Same as input
  Math Function1 : Math  Operator=sqrt  SignedPower=on
  Mux : Mux  Inputs=2
  Mux1 : Mux  Inputs=3
  Product : Product  InputSameDT=on  SaturateOnIntegerOverflow=on  OutDataTypeStr=Inherit: Same as first input
  Product1 : Product  InputSameDT=on  SaturateOnIntegerOverflow=on  OutDataTypeStr=Inherit: Same as first input
  Saturation : Saturate  UpperLimit=inf  LowerLimit=0
  Q : Outport  InitialOutput=0  VectorParamsAs1DForOutWhenUnconnected=off
  wires:
  u/1 -> Saturation/1
  dp/1 -> Fcn3/1, Fcn2/1
  Fcn/1 -> Mux1/3
  Mux/1 -> Fcn/1
  Product/1 -> Mux1/1
  Math Function1/1 -> Product/1
  Fcn3/1 -> Mux/1, Mux1/2, Math Function1/1
  Saturation/1 -> Gain/1
  Gain/1 -> Product/2, Mux/2
  Mux1/1 -> Fcn1/1
  Fcn1/1 -> Product1/2
  Fcn2/1 -> Product1/1
  Product1/1 -> Q/1

== system simulinkProject/Subsystem/4//3 Servovalve_4/Orifice P->A ==
  dp : Inport
  u : Inport  Port=2
  Fcn : Fcn  Expr=u[2]*u[1]/2.0/sqrt(ptr)*(3-u[1]/ptr)
  Fcn1 : Fcn  Expr=(u(2)>=ptr)*u(1)+(u(2)<ptr)*u(3)
  Fcn2 : Fcn  Expr=sgn(u(1))
  Fcn3 : Fcn  Expr=fabs(u(1))
  Gain : Gain  Gain=K  SaturateOnIntegerOverflow=on  OutDataTypeStr=Inherit: Same as input  ParamDataTypeStr=Inherit: Same as input
  Math Function1 : Math  Operator=sqrt  SignedPower=on
  Mux : Mux  Inputs=2
  Mux1 : Mux  Inputs=3
  Product : Product  InputSameDT=on  SaturateOnIntegerOverflow=on  OutDataTypeStr=Inherit: Same as first input
  Product1 : Product  InputSameDT=on  SaturateOnIntegerOverflow=on  OutDataTypeStr=Inherit: Same as first input
  Saturation : Saturate  UpperLimit=inf  LowerLimit=0
  Q : Outport  InitialOutput=0  VectorParamsAs1DForOutWhenUnconnected=off
  wires:
  u/1 -> Saturation/1
  dp/1 -> Fcn3/1, Fcn2/1
  Fcn/1 -> Mux1/3
  Mux/1 -> Fcn/1
  Product/1 -> Mux1/1
  Math Function1/1 -> Product/1
  Fcn3/1 -> Mux/1, Mux1/2, Math Function1/1
  Saturation/1 -> Gain/1
  Gain/1 -> Product/2, Mux/2
  Mux1/1 -> Fcn1/1
  Fcn1/1 -> Product1/2
  Fcn2/1 -> Product1/1
  Product1/1 -> Q/1

== system simulinkProject/Subsystem/4//3 Servovalve_4/Orifice P->B ==
  dp : Inport
  u : Inport  Port=2
  Fcn : Fcn  Expr=u[2]*u[1]/2.0/sqrt(ptr)*(3-u[1]/ptr)
  Fcn1 : Fcn  Expr=(u(2)>=ptr)*u(1)+(u(2)<ptr)*u(3)
  Fcn2 : Fcn  Expr=sgn(u(1))
  Fcn3 : Fcn  Expr=fabs(u(1))
  Gain : Gain  Gain=K  SaturateOnIntegerOverflow=on  OutDataTypeStr=Inherit: Same as input  ParamDataTypeStr=Inherit: Same as input
  Math Function1 : Math  Operator=sqrt  SignedPower=on
  Mux : Mux  Inputs=2
  Mux1 : Mux  Inputs=3
  Product : Product  InputSameDT=on  SaturateOnIntegerOverflow=on  OutDataTypeStr=Inherit: Same as first input
  Product1 : Product  InputSameDT=on  SaturateOnIntegerOverflow=on  OutDataTypeStr=Inherit: Same as first input
  Saturation : Saturate  UpperLimit=inf  LowerLimit=0
  Q : Outport  InitialOutput=0  VectorParamsAs1DForOutWhenUnconnected=off
  wires:
  u/1 -> Saturation/1
  dp/1 -> Fcn3/1, Fcn2/1
  Fcn/1 -> Mux1/3
  Mux/1 -> Fcn/1
  Product/1 -> Mux1/1
  Math Function1/1 -> Product/1
  Fcn3/1 -> Mux/1, Mux1/2, Math Function1/1
  Saturation/1 -> Gain/1
  Gain/1 -> Product/2, Mux/2
  Mux1/1 -> Fcn1/1
  Fcn1/1 -> Product1/2
  Fcn2/1 -> Product1/1
  Product1/1 -> Q/1

== system simulinkProject/Subsystem/4//3 Servovalve_4/Orifice T->A ==
  dp : Inport
  u : Inport  Port=2
  Fcn : Fcn  Expr=u[2]*u[1]/2.0/sqrt(ptr)*(3-u[1]/ptr)
  Fcn1 : Fcn  Expr=(u(2)>=ptr)*u(1)+(u(2)<ptr)*u(3)
  Fcn2 : Fcn  Expr=sgn(u(1))
  Fcn3 : Fcn  Expr=fabs(u(1))
  Gain : Gain  Gain=K  SaturateOnIntegerOverflow=on  OutDataTypeStr=Inherit: Same as input  ParamDataTypeStr=Inherit: Same as input
  Math Function1 : Math  Operator=sqrt  SignedPower=on
  Mux : Mux  Inputs=2
  Mux1 : Mux  Inputs=3
  Product : Product  InputSameDT=on  SaturateOnIntegerOverflow=on  OutDataTypeStr=Inherit: Same as first input
  Product1 : Product  InputSameDT=on  SaturateOnIntegerOverflow=on  OutDataTypeStr=Inherit: Same as first input
  Saturation : Saturate  UpperLimit=inf  LowerLimit=0
  Q : Outport  InitialOutput=0  VectorParamsAs1DForOutWhenUnconnected=off
  wires:
  u/1 -> Saturation/1
  dp/1 -> Fcn3/1, Fcn2/1
  Fcn/1 -> Mux1/3
  Mux/1 -> Fcn/1
  Product/1 -> Mux1/1
  Math Function1/1 -> Product/1
  Fcn3/1 -> Mux/1, Mux1/2, Math Function1/1
  Saturation/1 -> Gain/1
  Gain/1 -> Product/2, Mux/2
  Mux1/1 -> Fcn1/1
  Fcn1/1 -> Product1/2
  Fcn2/1 -> Product1/1
  Product1/1 -> Q/1

== system simulinkProject/Subsystem/4//3 Servovalve_4/Orifice T->B ==
  dp : Inport
  u : Inport  Port=2
  Fcn : Fcn  Expr=u[2]*u[1]/2.0/sqrt(ptr)*(3-u[1]/ptr)
  Fcn1 : Fcn  Expr=(u(2)>=ptr)*u(1)+(u(2)<ptr)*u(3)
  Fcn2 : Fcn  Expr=sgn(u(1))
  Fcn3 : Fcn  Expr=fabs(u(1))
  Gain : Gain  Gain=K  SaturateOnIntegerOverflow=on  OutDataTypeStr=Inherit: Same as input  ParamDataTypeStr=Inherit: Same as input
  Math Function1 : Math  Operator=sqrt  SignedPower=on
  Mux : Mux  Inputs=2
  Mux1 : Mux  Inputs=3
  Product : Product  InputSameDT=on  SaturateOnIntegerOverflow=on  OutDataTypeStr=Inherit: Same as first input
  Product1 : Product  InputSameDT=on  SaturateOnIntegerOverflow=on  OutDataTypeStr=Inherit: Same as first input
  Saturation : Saturate  UpperLimit=inf  LowerLimit=0
  Q : Outport  InitialOutput=0  VectorParamsAs1DForOutWhenUnconnected=off
  wires:
  u/1 -> Saturation/1
  dp/1 -> Fcn3/1, Fcn2/1
  Fcn/1 -> Mux1/3
  Mux/1 -> Fcn/1
  Product/1 -> Mux1/1
  Math Function1/1 -> Product/1
  Fcn3/1 -> Mux/1, Mux1/2, Math Function1/1
  Saturation/1 -> Gain/1
  Gain/1 -> Product/2, Mux/2
  Mux1/1 -> Fcn1/1
  Fcn1/1 -> Product1/2
  Fcn2/1 -> Product1/1
  Product1/1 -> Q/1

== system simulinkProject/Subsystem/Cylinder_1/Chamber A ==
  Net Flow : Inport
  " dV/dt" : Inport  Port=2
  " V" : Inport  Port=3
  " B" : Inport  Port=4
  Integrator : Integrator  InitialCondition=pinitial  LimitOutput=on  LowerSaturationLimit=0  AbsoluteTolerance=10
  Product : Product  Inputs=*/*  InputSameDT=on  SaturateOnIntegerOverflow=on  OutDataTypeStr=Inherit: Same as first input
  Sum : Sum  Inputs=+-  InputSameDT=on  SaturateOnIntegerOverflow=on  OutDataTypeStr=Inherit: Same as first input
  p : Outport  VectorParamsAs1DForOutWhenUnconnected=off
  wires:
  Product/1 -> Integrator/1
  " B"/1 -> Product/3
  " V"/1 -> Product/2
  Net Flow/1 -> Sum/1
  " dV/dt"/1 -> Sum/2
  Sum/1 -> Product/1
  Integrator/1 -> p/1

== system simulinkProject/Subsystem/Cylinder_1/Chamber B ==
  Net Flow : Inport
  " dV/dt" : Inport  Port=2
  " V" : Inport  Port=3
  " B" : Inport  Port=4
  Integrator : Integrator  InitialCondition=pinitial  LimitOutput=on  LowerSaturationLimit=0  AbsoluteTolerance=10
  Product : Product  Inputs=*/*  InputSameDT=on  SaturateOnIntegerOverflow=on  OutDataTypeStr=Inherit: Same as first input
  Sum : Sum  Inputs=+-  InputSameDT=on  SaturateOnIntegerOverflow=on  OutDataTypeStr=Inherit: Same as first input
  p : Outport  VectorParamsAs1DForOutWhenUnconnected=off
  wires:
  Product/1 -> Integrator/1
  " B"/1 -> Product/3
  " V"/1 -> Product/2
  Net Flow/1 -> Sum/1
  " dV/dt"/1 -> Sum/2
  Sum/1 -> Product/1
  Integrator/1 -> p/1

== system simulinkProject/Subsystem/Cylinder_2/Chamber A ==
  Net Flow : Inport
  " dV/dt" : Inport  Port=2
  " V" : Inport  Port=3
  " B" : Inport  Port=4
  Integrator : Integrator  InitialCondition=pinitial  LimitOutput=on  LowerSaturationLimit=0  AbsoluteTolerance=10
  Product : Product  Inputs=*/*  InputSameDT=on  SaturateOnIntegerOverflow=on  OutDataTypeStr=Inherit: Same as first input
  Sum : Sum  Inputs=+-  InputSameDT=on  SaturateOnIntegerOverflow=on  OutDataTypeStr=Inherit: Same as first input
  p : Outport  VectorParamsAs1DForOutWhenUnconnected=off
  wires:
  Product/1 -> Integrator/1
  " B"/1 -> Product/3
  " V"/1 -> Product/2
  Net Flow/1 -> Sum/1
  " dV/dt"/1 -> Sum/2
  Sum/1 -> Product/1
  Integrator/1 -> p/1

== system simulinkProject/Subsystem/Cylinder_2/Chamber B ==
  Net Flow : Inport
  " dV/dt" : Inport  Port=2
  " V" : Inport  Port=3
  " B" : Inport  Port=4
  Integrator : Integrator  InitialCondition=pinitial  LimitOutput=on  LowerSaturationLimit=0  AbsoluteTolerance=10
  Product : Product  Inputs=*/*  InputSameDT=on  SaturateOnIntegerOverflow=on  OutDataTypeStr=Inherit: Same as first input
  Sum : Sum  Inputs=+-  InputSameDT=on  SaturateOnIntegerOverflow=on  OutDataTypeStr=Inherit: Same as first input
  p : Outport  VectorParamsAs1DForOutWhenUnconnected=off
  wires:
  Product/1 -> Integrator/1
  " B"/1 -> Product/3
  " V"/1 -> Product/2
  Net Flow/1 -> Sum/1
  " dV/dt"/1 -> Sum/2
  Sum/1 -> Product/1
  Integrator/1 -> p/1

== system simulinkProject/Subsystem/Cylinder_3/Chamber A ==
  Net Flow : Inport
  " dV/dt" : Inport  Port=2
  " V" : Inport  Port=3
  " B" : Inport  Port=4
  Integrator : Integrator  InitialCondition=pinitial  LimitOutput=on  LowerSaturationLimit=0  AbsoluteTolerance=10
  Product : Product  Inputs=*/*  InputSameDT=on  SaturateOnIntegerOverflow=on  OutDataTypeStr=Inherit: Same as first input
  Sum : Sum  Inputs=+-  InputSameDT=on  SaturateOnIntegerOverflow=on  OutDataTypeStr=Inherit: Same as first input
  p : Outport  VectorParamsAs1DForOutWhenUnconnected=off
  wires:
  Product/1 -> Integrator/1
  " B"/1 -> Product/3
  " V"/1 -> Product/2
  Net Flow/1 -> Sum/1
  " dV/dt"/1 -> Sum/2
  Sum/1 -> Product/1
  Integrator/1 -> p/1

== system simulinkProject/Subsystem/Cylinder_3/Chamber B ==
  Net Flow : Inport
  " dV/dt" : Inport  Port=2
  " V" : Inport  Port=3
  " B" : Inport  Port=4
  Integrator : Integrator  InitialCondition=pinitial  LimitOutput=on  LowerSaturationLimit=0  AbsoluteTolerance=10
  Product : Product  Inputs=*/*  InputSameDT=on  SaturateOnIntegerOverflow=on  OutDataTypeStr=Inherit: Same as first input
  Sum : Sum  Inputs=+-  InputSameDT=on  SaturateOnIntegerOverflow=on  OutDataTypeStr=Inherit: Same as first input
  p : Outport  VectorParamsAs1DForOutWhenUnconnected=off
  wires:
  Product/1 -> Integrator/1
  " B"/1 -> Product/3
  " V"/1 -> Product/2
  Net Flow/1 -> Sum/1
  " dV/dt"/1 -> Sum/2
  Sum/1 -> Product/1
  Integrator/1 -> p/1

== system simulinkProject/Subsystem/Cylinder_4/Chamber A ==
  Net Flow : Inport
  " dV/dt" : Inport  Port=2
  " V" : Inport  Port=3
  " B" : Inport  Port=4
  Integrator : Integrator  InitialCondition=pinitial  LimitOutput=on  LowerSaturationLimit=0  AbsoluteTolerance=10
  Product : Product  Inputs=*/*  InputSameDT=on  SaturateOnIntegerOverflow=on  OutDataTypeStr=Inherit: Same as first input
  Sum : Sum  Inputs=+-  InputSameDT=on  SaturateOnIntegerOverflow=on  OutDataTypeStr=Inherit: Same as first input
  p : Outport  VectorParamsAs1DForOutWhenUnconnected=off
  wires:
  Product/1 -> Integrator/1
  " B"/1 -> Product/3
  " V"/1 -> Product/2
  Net Flow/1 -> Sum/1
  " dV/dt"/1 -> Sum/2
  Sum/1 -> Product/1
  Integrator/1 -> p/1

== system simulinkProject/Subsystem/Cylinder_4/Chamber B ==
  Net Flow : Inport
  " dV/dt" : Inport  Port=2
  " V" : Inport  Port=3
  " B" : Inport  Port=4
  Integrator : Integrator  InitialCondition=pinitial  LimitOutput=on  LowerSaturationLimit=0  AbsoluteTolerance=10
  Product : Product  Inputs=*/*  InputSameDT=on  SaturateOnIntegerOverflow=on  OutDataTypeStr=Inherit: Same as first input
  Sum : Sum  Inputs=+-  InputSameDT=on  SaturateOnIntegerOverflow=on  OutDataTypeStr=Inherit: Same as first input
  p : Outport  VectorParamsAs1DForOutWhenUnconnected=off
  wires:
  Product/1 -> Integrator/1
  " B"/1 -> Product/3
  " V"/1 -> Product/2
  Net Flow/1 -> Sum/1
  " dV/dt"/1 -> Sum/2
  Sum/1 -> Product/1
  Integrator/1 -> p/1
